simulink model "SimulatedNetworkModel"  (R2024b)
settings: Solver=VariableStepAuto  StartTime=0.0  StopTime=10.0  RelTol=1e-3
libraries: ee_lib x7, fl_lib x6, nesl_utility x1
settings Model: Creator=xinxing  LastModifiedBy=xinxing

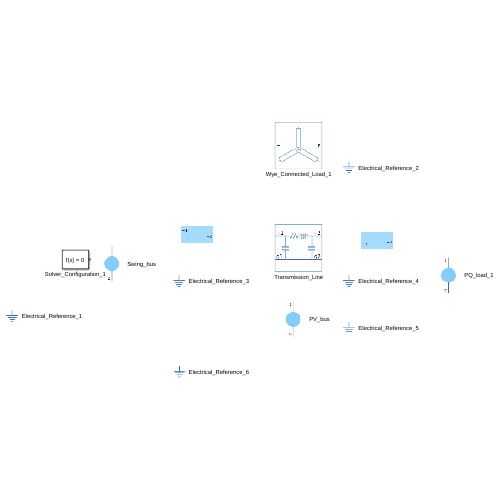
[thumbnail: Simulink's stored preview of the top-level diagram]
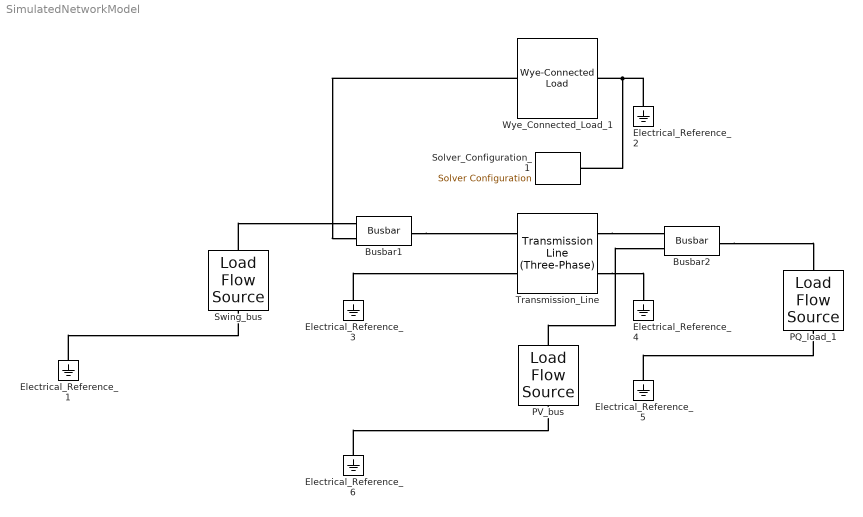
== system SimulatedNetworkModel ==
  Busbar1 : ee_lib/Connectors & References/Busbar  n_nodes=3  VRated=sqrt(3) * 100 / sqrt(2) V  freq=60 Hz  show_ps=ee.enum.connectors.busbar_measurement.false
      settings: AttributesFormatString=%<Tag>  InternalSimscapePortConfiguration="{\"Bottom\":[],\"Left\":[{\"id\":\"N1\",\"label\":\"~1\",\"type\":\"foundation.electrical.three_phase\"},{\"id\":\"N3\",\"label\":\"~3\",\"type\":\"foundation.electrical.three_phase\"}],\"Right\":[{\"id\":\"N2\",\"label\":\"~2\",\"type\":\"foundation.electrical.three_phase\"}],\"Top\":[]}"
  Busbar2 : ee_lib/Connectors & References/Busbar  n_nodes=3  VRated=sqrt(3) * 100 / sqrt(2) V  freq=60 Hz  show_ps=ee.enum.connectors.busbar_measurement.false
      settings: AttributesFormatString=%<Tag>  InternalSimscapePortConfiguration="{\"Bottom\":[],\"Left\":[{\"id\":\"N1\",\"label\":\"~1\",\"type\":\"foundation.electrical.three_phase\"},{\"id\":\"N3\",\"label\":\"~3\",\"type\":\"foundation.electrical.three_phase\"}],\"Right\":[{\"id\":\"N2\",\"label\":\"~2\",\"type\":\"foundation.electrical.three_phase\"}],\"Top\":[]}"
  Electrical_Reference_{1..6} (6 alike) : fl_lib/Electrical/Electrical Elements/Electrical Reference
  PQ_load_1 : ee_lib/Sources/Load Flow Source  source_type=ee.enum.sources.load_flow_source_type.Swing  v_pu_src=1  active_power_generated=0 W  active_power_consumed=0 W  reactive_power_consumed=0 A*V  v_pu=1  VRated=sqrt(3) * 100 / sqrt(2) V  freq=60 Hz  shift_src=0 deg  impedance_option=ee.enum.sources.load_flow_source_impedance.None  SShortCircuit=1e6 A*V  XR=15  R=0.01 Ohm  L=3.97e-4 H  G_parasitic=0 1/Ohm  minimum_pu=0.95  phase_search_range=[-inf, inf] deg  I_specify=off  I_priority=None  I=[0, 0, 0] A  I_nominal_specify=off  I_nominal_value=1  I_nominal_unit=A  V_impedance_specify=off  V_impedance_priority=None  V_impedance=[0, 0, 0] V  V_impedance_nominal_specify=off  V_impedance_nominal_value=1  V_impedance_nominal_unit=V
      settings: InternalSimscapePortConfiguration="{\"Bottom\":[],\"Left\":[{\"id\":\"N\",\"label\":\"~\",\"type\":\"foundation.electrical.three_phase\"}],\"Right\":[{\"id\":\"n\",\"label\":\"n\",\"type\":\"foundation.electrical.electrical\"}],\"Top\":[]}"
  PV_bus : ee_lib/Sources/Load Flow Source  source_type=ee.enum.sources.load_flow_source_type.Swing  v_pu_src=1  active_power_generated=0 W  active_power_consumed=0 W  reactive_power_consumed=0 A*V  v_pu=1  VRated=sqrt(3) * 100 / sqrt(2) V  freq=60 Hz  shift_src=0 deg  impedance_option=ee.enum.sources.load_flow_source_impedance.None  SShortCircuit=1e6 A*V  XR=15  R=0.01 Ohm  L=3.97e-4 H  G_parasitic=0 1/Ohm  minimum_pu=0.95  phase_search_range=[-inf, inf] deg  I_specify=off  I_priority=None  I=[0, 0, 0] A  I_nominal_specify=off  I_nominal_value=1  I_nominal_unit=A  V_impedance_specify=off  V_impedance_priority=None  V_impedance=[0, 0, 0] V  V_impedance_nominal_specify=off  V_impedance_nominal_value=1  V_impedance_nominal_unit=V
      settings: InternalSimscapePortConfiguration="{\"Bottom\":[],\"Left\":[{\"id\":\"N\",\"label\":\"~\",\"type\":\"foundation.electrical.three_phase\"}],\"Right\":[{\"id\":\"n\",\"label\":\"n\",\"type\":\"foundation.electrical.electrical\"}],\"Top\":[]}"
  Solver_Configuration_1 : nesl_utility/Solver Configuration  PhysicalDomain=network_engine_domain  SubClassName=solver  LeftPortType=input  RightPortType=generic  Tones=[]  Harmonics=[]  SimulateNoise=off  Profile=off  UseLocalSampling=off  EnableSwitchedLinearOptims=on  FrequencyDomain=off  UseCCode=off  RelTol=0.001  AbsTol=0.001  MinStep=1e-09  ToWorkspace=off  RevertToSquareIcSolve=off  NumHomotopyIterations=100  PhasorMode=off  PhasorModeNumHarmonics=1  ConsistencySolver=NEWTON_XTOL_AFTER_FTOL  IndexReductionMethod=DerivativeReplacement  DoDC=off  ResidualTolerance=1e-09  ConsistencyTolSource=GLOBAL  ConsistencyAbsTol=0.001  ConsistencyRelTol=0.001  ConsistencyTolFactor=0.001  UseLocalSolver=off  LocalSolverChoice=NE_BACKWARD_EULER_ADVANCER  ResolveIndetEquations=on  FunctionEvalNumThread=1  LocalSolverSampleTime=0.001  DoFixedCost=off  MaxNonlinIter=3  MaxModeIter=2  ComputeImpulses=off  ImpulseIterations=2  LinearAlgebra=auto  LinearAlgebraNumThread=0  EquationFormulation=NE_TIME_EF  DelaysMemoryBudget=1024  AutomaticFiltering=on  FilteringTimeConstant=0.001  PartitionStorageMethod=AS_NEEDED  PartitionMemoryBudget=1024  PartitionMethod=ROBUST  MultibodyUseLocalSolver=off  MultibodyLocalSolverChoice=ODE1  MultibodyLocalSolverSampleTime=0.001
  Swing_bus : ee_lib/Sources/Load Flow Source  source_type=ee.enum.sources.load_flow_source_type.Swing  v_pu_src=1  active_power_generated=0 W  active_power_consumed=0 W  reactive_power_consumed=0 A*V  v_pu=1  VRated=sqrt(3) * 100 / sqrt(2) V  freq=60 Hz  shift_src=0 deg  impedance_option=ee.enum.sources.load_flow_source_impedance.None  SShortCircuit=1e6 A*V  XR=15  R=0.01 Ohm  L=3.97e-4 H  G_parasitic=0 1/Ohm  minimum_pu=0.95  phase_search_range=[-inf, inf] deg  I_specify=off  I_priority=None  I=[0, 0, 0] A  I_nominal_specify=off  I_nominal_value=1  I_nominal_unit=A  V_impedance_specify=off  V_impedance_priority=None  V_impedance=[0, 0, 0] V  V_impedance_nominal_specify=off  V_impedance_nominal_value=1  V_impedance_nominal_unit=V
      settings: InternalSimscapePortConfiguration="{\"Bottom\":[],\"Left\":[{\"id\":\"N\",\"label\":\"~\",\"type\":\"foundation.electrical.three_phase\"}],\"Right\":[{\"id\":\"n\",\"label\":\"n\",\"type\":\"foundation.electrical.electrical\"}],\"Top\":[]}"
  Transmission_Line : ee_lib/Passive/Lines/Transmission Line (Three-Phase)  length=1 km  freq=60 Hz  R=0.02 Ohm/km  L=0.5 mH/km  M=0.1 mH/km  Cl=0.3 uF/km  Cg=0.1 uF/km  Rm=0 Ohm/km  ModelTwoSections=ee.enum.enable.no  N=1  InterfacePosition=0.5 km  N1sec=1  N2sec=1  Access_ground=ee.enum.enable.no  R_parasitic=1e-6 Ohm  G_parasitic=1e-6 1/Ohm
      settings: InternalSimscapePortConfiguration="{\"Bottom\":[],\"Left\":[{\"id\":\"N1\",\"label\":\"~1\",\"type\":\"foundation.electrical.three_phase\"},{\"id\":\"g1\",\"label\":\"g1\",\"type\":\"foundation.electrical.electrical\"}],\"Right\":[{\"id\":\"N2\",\"label\":\"~2\",\"type\":\"foundation.electrical.three_phase\"},{\"id\":\"g2\",\"label\":\"g2\",\"type\":\"foundation.electrical.electrical\"}],\"Top\":[]}"
  Wye_Connected_Load_1 : ee_lib/Passive/RLC Assemblies/Wye-Connected Load  port_option=ee.enum.threePhasePort.composite  parameterization=ee.enum.rlc.parameterization.ratedpower  component_structure=ee.enum.rlc.structure.R  component_structure_PQ=ee.enum.rlc.structure.R  R=1 Ohm  L=1e-3 H  C=1e-6 F  VRated=24e3 V  FRated=60 Hz  P=1e3 W  Qpos=1e2 A*V  Qneg=-1e2 A*V  R_parasitic=1e-6 Ohm  G_parasitic=1e-6 1/Ohm  R_parasitic_PQ=1e-6 Ohm  G_parasitic_PQ=1e-6 1/Ohm  Vmag0=24e3 V  Vang0=0 deg  Freq0=60 Hz  IL_specify=off  IL_priority=High  IL=[0, 0, 0] A  IL_nominal_specify=off  IL_nominal_value=1  IL_nominal_unit=A  VC_specify=off  VC_priority=High  VC=[0, 0, 0] V  VC_nominal_specify=off  VC_nominal_value=1  VC_nominal_unit=V
  connections:
  Electrical_Reference_5/LConn1 -- PQ_load_1/RConn1
  Electrical_Reference_2/LConn1 -- Wye_Connected_Load_1/RConn1 -- Solver_Configuration_1/RConn1
  Transmission_Line/RConn2 -- Electrical_Reference_4/LConn1
  Busbar2/RConn1 -- PQ_load_1/LConn1
  Transmission_Line/RConn1 -- Busbar2/LConn1
  Wye_Connected_Load_1/LConn1 -- Busbar1/LConn2
  PV_bus/LConn1 -- Busbar2/LConn2
  Electrical_Reference_6/LConn1 -- PV_bus/RConn1
  Electrical_Reference_3/LConn1 -- Transmission_Line/LConn2
  Busbar1/RConn1 -- Transmission_Line/LConn1
  Swing_bus/LConn1 -- Busbar1/LConn1
  Electrical_Reference_1/LConn1 -- Swing_bus/RConn1
